simulink model "ex2_6_sim"  (R2022b)
settings: Solver=VariableStepAuto  StartTime=0.0  StopTime=T_stop  RelTol=1e-3
values from neighbouring files (symbols this model uses):
  C = Cp*m    (= 75831.7634724)    [ex2_6.m]
  Rconv = 1/(A*h)    (= 3.18309886184)    [ex2_6.m]    (also in ex2_7_cstes.m = 6.36619772368)
  Ta = 100    [ex2_6.m]
  Tb = 10    [ex2_6.m]
  Tint0 = 25    [ex2_6.m]
settings Model: Creator=nicol  LastModifiedBy=nicol

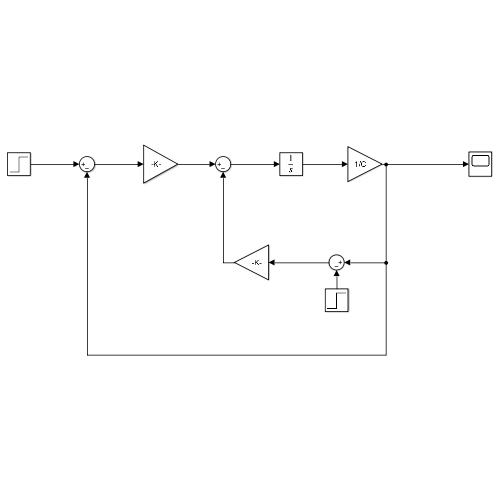
[thumbnail: Simulink's stored preview of the top-level diagram]
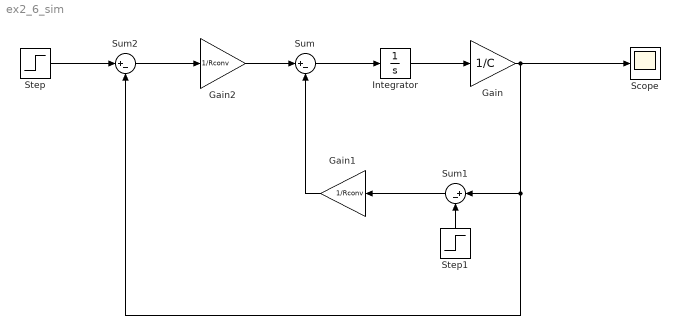
== system ex2_6_sim ==
  Gain : Gain  Gain=1/C
  Gain1 : Gain  Gain=1/Rconv
  Gain2 : Gain  Gain=1/Rconv
  Integrator : Integrator  InitialCondition=Tint0*C
  Scope : Scope
  Step : Step  Time=0  After=Ta  SampleTime=0
  Step1 : Step  Time=0  After=Tb  SampleTime=0
  Sum : Sum  Inputs=|+-
  Sum1 : Sum  Inputs=|+-
  Sum2 : Sum  Inputs=|+-
  wires:
  Gain/1 -> Sum2/2, Sum1/1, Scope/1
  Sum1/1 -> Gain1/1
  Gain1/1 -> Sum/2
  Sum2/1 -> Gain2/1
  Gain2/1 -> Sum/1
  Sum/1 -> Integrator/1
  Integrator/1 -> Gain/1
  Step/1 -> Sum2/1
  Step1/1 -> Sum1/2
